simulink model "SC228_TrackedRadarModelUnitTest"  (R2018b)
settings: Solver=VariableStepAuto  StartTime=0.0  StopTime=180  RelTol=1e-3
model workspace (MAT data in the model file):
  E_tracked_bias_stddev_ft = Simulink.Parameter
  E_tracked_bias_stddev_ft.Value = 0
  E_tracked_bias_stddev_ft.DataType = 'auto'
  E_tracked_bias_stddev_ft.Dimensions = [1 1]
  E_tracked_random_stddev_ft = Simulink.Parameter
  E_tracked_random_stddev_ft.Value = 250
  E_tracked_random_stddev_ft.DataType = 'auto'
  E_tracked_random_stddev_ft.Dimensions = [1 1]
  Edot_tracked_bias_stddev_ftps = Simulink.Parameter
  Edot_tracked_bias_stddev_ftps.Value = 0
  Edot_tracked_bias_stddev_ftps.DataType = 'auto'
  Edot_tracked_bias_stddev_ftps.Dimensions = [1 1]
  Edot_tracked_random_stddev_ftps = Simulink.Parameter
  Edot_tracked_random_stddev_ftps.Value = 84.3904928551
  Edot_tracked_random_stddev_ftps.DataType = 'auto'
  Edot_tracked_random_stddev_ftps.Dimensions = [1 1]
  Edot_tracked_tau_s = Simulink.Parameter
  Edot_tracked_tau_s.Value = 0
  Edot_tracked_tau_s.DataType = 'auto'
  Edot_tracked_tau_s.Dimensions = [1 1]
  N_tracked_bias_stddev_ft = Simulink.Parameter
  N_tracked_bias_stddev_ft.Value = 0
  N_tracked_bias_stddev_ft.DataType = 'auto'
  N_tracked_bias_stddev_ft.Dimensions = [1 1]
  N_tracked_random_stddev_ft = 250
  N_tracked_tau_s = Simulink.Parameter
  N_tracked_tau_s.Value = 0
  N_tracked_tau_s.DataType = 'auto'
  N_tracked_tau_s.Dimensions = [1 1]
  Ndot_tracked_bias_stddev_ftps = Simulink.Parameter
  Ndot_tracked_bias_stddev_ftps.Value = 0
  Ndot_tracked_bias_stddev_ftps.DataType = 'auto'
  Ndot_tracked_bias_stddev_ftps.Dimensions = [1 1]
  Ndot_tracked_random_stddev_ftps = Simulink.Parameter
  Ndot_tracked_random_stddev_ftps.Value = 84.3904928551
  Ndot_tracked_random_stddev_ftps.DataType = 'auto'
  Ndot_tracked_random_stddev_ftps.Dimensions = [1 1]
  Ndot_tracked_tau_s = Simulink.Parameter
  Ndot_tracked_tau_s.Value = 0
  Ndot_tracked_tau_s.DataType = 'auto'
  Ndot_tracked_tau_s.Dimensions = [1 1]
  tracked_az_bias_rad = Simulink.Parameter
  tracked_az_bias_rad.Value = 0
  tracked_az_bias_rad.DataType = 'auto'
  tracked_az_bias_rad.Dimensions = [1 1]
  tracked_az_random_stddev_rad = Simulink.Parameter
  tracked_az_random_stddev_rad.Value = 0.0174532925199
  tracked_az_random_stddev_rad.DataType = 'auto'
  tracked_az_random_stddev_rad.Dimensions = [1 1]
  tracked_rng_bias_ft = Simulink.Parameter
  tracked_rng_bias_ft.DataType = 'auto'
  tracked_rng_bias_ft.Dimensions = [0 0]
undefined symbols (not defined in the file or in its folder): ac1dyn_alt0_ft, ac1dyn_con, ac1dyn_lat0_rad, ac1dyn_lon0_rad, ac2dyn_alt0_ft, ac2dyn_con, ac2dyn_lat0_rad, ac2dyn_lon0_rad, ddh_ftps2, dh_ftps, dv_ftps2, e_ft, Edot_ftps, h_ft, hdot_ftps, latLonAltState, n_ft, Ndot_ftps, p_radps, phi_rad, phidot_radps, psi_rad, psidot_radps, q_radps, r_radps, theta_rad, thetadot_radps, uas_rdr_trckd_az_bias_ft, uas_rdr_trckd_az_bias_rad, uas_rdr_trckd_az_random_stddev_rad, uas_rdr_trckd_az_stddev_ft, uas_rdr_trckd_azdot_bias_ftps, uas_rdr_trckd_azdot_stddev_ftps, uas_rdr_trckd_debugMode, uas_rdr_trckd_dt_s, uas_rdr_trckd_el_bias_ft, uas_rdr_trckd_el_bias_rad, uas_rdr_trckd_el_random_stddev_rad, uas_rdr_trckd_el_stddev_ft, uas_rdr_trckd_eldot_bias_ftps, uas_rdr_trckd_eldot_stddev_ftps, uas_rdr_trckd_RCPR_Mode, uas_rdr_trckd_RCPR_Range_ft, uas_rdr_trckd_reported_errorCovRAE, uas_rdr_trckd_rng_bias_ft, uas_rdr_trckd_rng_random_stddev_ft, uas_rdr_trckd_rngdot_bias_ftps, uas_rdr_trckd_rngdot_random_stddev_ftps, uas_rdr_trckd_seed1, uas_rdr_trckd_seed2, uas_rdr_trckd_seed3, uas_rdr_trckd_seed4, uas_rdr_trckd_sns_for_azimuth_deg, uas_rdr_trckd_sns_for_elevation_deg, v_ftps, vdot_fpss
libraries: simulink x17, dspmtrx3 x1
(part 1 of 2)
settings Model: Creator=PE29732  LastModifiedBy=PE29732

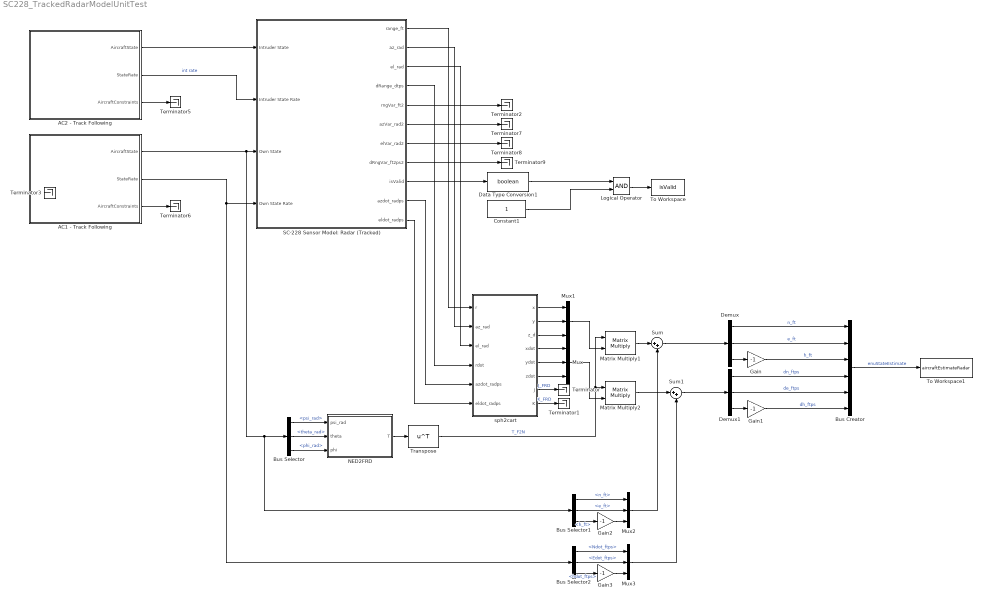
== system SC228_TrackedRadarModelUnitTest ==
  AC1 - Track Following : Subsystem  mask(Basic Aircraft Dynamic Model){ts_dynamics=0.1, lat0_rad=ac1dyn_lat0_rad, lon0_rad=ac1dyn_lon0_rad, alt_ft=ac1dyn_alt0_ft, v_ftps_max=ac1dyn_con.maxAirspeed_ftps, v_ftps_min=ac1dyn_con.minAirspeed_ftps, dv_ftpss_max=ac1dyn_con.maxAcceleration_ftpss, dv_ftpss_min=ac1dyn_con.minAcceleration_ftpss, dh_ftps_max=ac1dyn_con.maxVerticalRate_ftps, dh_ftps_min=ac1dyn_con.minVerticalRate_ftps, q_radps_max=ac1dyn_con.maxPitchRate_radps, phi_rad_max=ac1dyn_con.maxBankAngle_rad, dphi_radps_max=ac1dyn_con.maxRollRate_radps, r_radps_max=ac1dyn_con.maxYawRate_radps, pNUM=ac1dyn_con.dynamicsNumeratorRollRate, pDEN=ac1dyn_con.dynamicsDenominatorRollRate, hNUM=ac1dyn_con.dynamicsNumeratorVerticalRate, hDEN=ac1dyn_con.dynamicsDenominatorVerticalRate, rNUM=ac1dyn_con.dynamicsNumeratorYawRate, rDEN=ac1dyn_con.dynamicsDenominatorYawRate}
      mask prompts: ts_dynamics "Dynamics update parameter"; lat0_rad "Latitude of ENU origin (rad)"; lon0_rad "Longitude of ENU origin (rad)"; alt_ft "Height of ENU origin (ft)"; v_ftps_max "Maximum airspeed (ft/s)"; v_ftps_min "Minimum airspeed (ft/s)"; dv_ftpss_max "Maximum acceleration (ft/s/s)"; dv_ftpss_min "Miniimum acceleration (ft/s/s)"; dh_ftps_max "Maximum vertical rate (ft/s)"; dh_ftps_min "Minimum vertical rate (ft/s)"; q_radps_max "Maximum pitch rate (rad/s)"; phi_rad_max "Maximum bank angle (rad)"; dphi_radps_max "Maximum roll rate (rad/s)"; r_radps_max "Maximum yaw rate (rad/s)"; pNUM "Roll rate discrete dynamics numerator (2x1)"; pDEN "Roll rate discrete dynamics denominator (1x1)"; hNUM "Vertical rate discrete dynamics numerator (2x1)"; hDEN "Vertical rate discrete dynamics denominator (1x1)"; rNUM "Yaw rate discrete dynamics numerator (2x1)"; rDEN "Yaw rate discrete dynamics denominator (1x1)"
      mask help:
      | Propagates the aircraft dynamics using 6DOF equations of motion.
      |
      | The class Simple6DOF can be used to programmatically set the parameters of Basic Aircraft Dynamcis blocks.
      mask Help:
      | Propagates the aircraft dynamics using 6DOF equations of motion.
      | 
      | The class Simple6DOF can be used to programmatically set the parameters of Basic Aircraft Dynamcis blocks.
      mask DialogControl ParameterTabVar0 Prompt: Main
      mask DialogControl ParameterTabVar01 Prompt: Constraints
  AC2 - Track Following : Subsystem  mask(Basic Aircraft Dynamic Model){ts_dynamics=0.1, lat0_rad=ac2dyn_lat0_rad, lon0_rad=ac2dyn_lon0_rad, alt_ft=ac2dyn_alt0_ft, v_ftps_max=ac2dyn_con.maxAirspeed_ftps, v_ftps_min=ac2dyn_con.minAirspeed_ftps, dv_ftpss_max=ac2dyn_con.maxAcceleration_ftpss, dv_ftpss_min=ac2dyn_con.minAcceleration_ftpss, dh_ftps_max=ac2dyn_con.maxVerticalRate_ftps, dh_ftps_min=ac2dyn_con.minVerticalRate_ftps, q_radps_max=ac2dyn_con.maxPitchRate_radps, phi_rad_max=ac2dyn_con.maxBankAngle_rad, dphi_radps_max=ac2dyn_con.maxRollRate_radps, r_radps_max=ac2dyn_con.maxYawRate_radps, pNUM=ac2dyn_con.dynamicsNumeratorRollRate, pDEN=ac2dyn_con.dynamicsDenominatorRollRate, hNUM=ac2dyn_con.dynamicsNumeratorVerticalRate, hDEN=ac2dyn_con.dynamicsDenominatorVerticalRate, rNUM=ac2dyn_con.dynamicsNumeratorYawRate, rDEN=ac2dyn_con.dynamicsDenominatorYawRate}
      mask prompts: ts_dynamics "Dynamics update parameter"; lat0_rad "Latitude of ENU origin (rad)"; lon0_rad "Longitude of ENU origin (rad)"; alt_ft "Height of ENU origin (ft)"; v_ftps_max "Maximum airspeed (ft/s)"; v_ftps_min "Minimum airspeed (ft/s)"; dv_ftpss_max "Maximum acceleration (ft/s/s)"; dv_ftpss_min "Miniimum acceleration (ft/s/s)"; dh_ftps_max "Maximum vertical rate (ft/s)"; dh_ftps_min "Minimum vertical rate (ft/s)"; q_radps_max "Maximum pitch rate (rad/s)"; phi_rad_max "Maximum bank angle (rad)"; dphi_radps_max "Maximum roll rate (rad/s)"; r_radps_max "Maximum yaw rate (rad/s)"; pNUM "Roll rate discrete dynamics numerator (2x1)"; pDEN "Roll rate discrete dynamics denominator (1x1)"; hNUM "Vertical rate discrete dynamics numerator (2x1)"; hDEN "Vertical rate discrete dynamics denominator (1x1)"; rNUM "Yaw rate discrete dynamics numerator (2x1)"; rDEN "Yaw rate discrete dynamics denominator (1x1)"
      mask help:
      | Propagates the aircraft dynamics using 6DOF equations of motion.
      |
      | The class Simple6DOF can be used to programmatically set the parameters of Basic Aircraft Dynamcis blocks.
      mask Help:
      | Propagates the aircraft dynamics using 6DOF equations of motion.
      | 
      | The class Simple6DOF can be used to programmatically set the parameters of Basic Aircraft Dynamcis blocks.
      mask DialogControl ParameterTabVar0 Prompt: Main
      mask DialogControl ParameterTabVar01 Prompt: Constraints
  Bus Creator : BusCreator  Inputs=6  OutDataTypeStr=Bus: StateEstimate
  Bus Selector : BusSelector  OutputSignals=psi_rad,theta_rad,phi_rad
  Bus Selector1 : BusSelector  OutputSignals=n_ft,e_ft,h_ft
  Bus Selector2 : BusSelector  OutputSignals=Ndot_ftps,Edot_ftps,hdot_ftps
  Constant1 : Constant
  Data Type Conversion1 : DataTypeConversion  OutDataTypeStr=boolean
  Demux : Demux  Outputs=3
  Demux1 : Demux  Outputs=3
  Gain{,1..3} (4 alike) : Gain  Gain=-1
  Logical Operator : Logic  AllPortsSameDT=off  OutDataTypeStr=boolean
  Matrix Multiply1 : Product  Multiplication=Matrix(*)
  Matrix Multiply2 : Product  Multiplication=Matrix(*)
  Mux{,1..3} (4 alike) : Mux  Inputs=3
  NED2FRD : MATLAB Function  TreatAsAtomicUnit=on
  SC-228 Sensor Model: Radar (Tracked) : Subsystem  mask(Tracked Surveillance: Radar){dt_s=uas_rdr_trckd_dt_s, lat0_rad=ac1dyn_lat0_rad, lon0_rad=ac1dyn_lon0_rad, alt0_ft=ac1dyn_alt0_ft, sns_for_azimuth_deg=uas_rdr_trckd_sns_for_azimuth_deg, sns_for_elevation_deg=uas_rdr_trckd_sns_for_elevation_deg, debugMode=uas_rdr_trckd_debugMode, rng_random_stddev_ft=uas_rdr_trckd_rng_random_stddev_ft, rng_bias_ft=uas_rdr_trckd_rng_bias_ft, rng_tau_s=0, seed1=uas_rdr_trckd_seed1, RCPR_Mode=uas_rdr_trckd_RCPR_Mode, RCPR_Range_ft=uas_rdr_trckd_RCPR_Range_ft, az_random_stddev_rad=uas_rdr_trckd_az_random_stddev_rad, az_bias_rad=uas_rdr_trckd_az_bias_rad, az_tau_s=0, seed2=uas_rdr_trckd_seed2, el_random_stddev_rad=uas_rdr_trckd_el_random_stddev_rad, el_bias_rad=uas_rdr_trckd_el_bias_rad, el_tau_s=0, seed3=uas_rdr_trckd_seed3, rngdot_random_stddev_ftps=uas_rdr_trckd_rngdot_random_stddev_ftps, rngdot_bias_ftps=uas_rdr_trckd_rngdot_bias_ftps, rngdot_tau_s=0, seed4=uas_rdr_trckd_seed4, covRAE=uas_rdr_trckd_reported_errorCovRAE}
      mask prompts: dt_s "Timestep"; lat0_rad "ENU Origin Latitude"; lon0_rad "ENU Origin Longitude"; alt0_ft "ENU Origin Altitude"; sns_for_azimuth_deg "Field of Regard: Azimuth Limit (deg)"; sns_for_elevation_deg "Field of Regard: Elevation Limit (deg)"; debugMode "Whether to run in debug mode with inifinite detection range"; rng_random_stddev_ft "Range Random Error Standard Deviation"; rng_bias_ft "Range Bias"; rng_tau_s "Correlation Time"; seed1 "Random Seed"; RCPR_Mode "RCPR Mode (1 = minimum range enabled, 0 = not enabled)"; RCPR_Range_ft "RCPR Range (ft)"; az_random_stddev_rad "Azimuth Random Error Standard Deviation"; az_bias_rad "Azimuth Bias"; az_tau_s "Correlation Time"; seed2 "Random Seed"; el_random_stddev_rad "Elevation Random Error Standard Deviation"; el_bias_rad "Elevation Bias"; el_tau_s "Correlation Time"; seed3 "Random Seed"; rngdot_random_stddev_ftps "Range Rate Random Error Standard Deviation"; rngdot_bias_ftps "Range Rate Bias"; rngdot_tau_s "Correlation Time"; seed4 "Random Seed"; covRAE "Error Covariance"
      mask help: Additive noise model of an on-board radar
      mask Help:
      | Additive noise model of an on-board radar.  Independent noise is added to
      | each of range, azimuth, elevation and their rates.  Noise is colored using
      | weights determined by time constant parameters.
      | 
      | Output takes the form of a AircraftEstimate data bus and a 6x6 error covariance
      | matrix in North-East-Down.  State order in error covariance output is
      | [ posN posE posD velN velE velD ].
      | 
      | Model originally developed for USAF Common ABSAA Program Nov 2013
      mask DialogControl ParameterTabVar0 Prompt: Tab
      mask DialogControl ParameterTabVar01 Prompt: Range
      mask DialogControl ParameterTabVar012 Prompt: Azimuth
      mask DialogControl ParameterTabVar0123 Prompt: Elevation
      mask DialogControl ParameterTabVar01234 Prompt: Range rate
      mask DialogControl ParameterTabVar01234567 Prompt: Covariance
  Sum : Sum  Inputs=|++
  Sum1 : Sum  Inputs=|++
  Terminator{,1..3,5..9} (9 alike) : Terminator
  To Workspace : ToWorkspace  VariableName=isValid  SaveFormat=Timeseries  SampleTime=-1
  To Workspace1 : ToWorkspace  VariableName=aircraftEstimateRadar  SaveFormat=Timeseries  SampleTime=-1
  Transpose : Math  Operator=transpose  SaturateOnIntegerOverflow=on
  sph2cart : MATLAB Function  TreatAsAtomicUnit=on
  wires:
  AC1 - Track Following/2(StateRate) -> Bus Selector2/1, SC-228 Sensor Model: Radar (Tracked)/4(Own State Rate)
  Bus Selector2/1 -> Mux3/1  "<Ndot_ftps>"
  Data Type Conversion1/1 -> Logical Operator/1
  SC-228 Sensor Model: Radar (Tracked)/10(azdot_radps) -> sph2cart/5(azdot_radps)
  sph2cart/1(x) -> Mux1/1
  Bus Creator/1 -> To Workspace1/1  "enuStateEstimate"
  AC2 - Track Following/1(AircraftState) -> SC-228 Sensor Model: Radar (Tracked)/1(Intruder State)
  Gain1/1 -> Bus Creator/6  "dh_ftps"
  SC-228 Sensor Model: Radar (Tracked)/2(az_rad) -> sph2cart/2(az_rad)
  Gain/1 -> Bus Creator/3  "h_ft"
  Bus Selector1/3 -> Gain2/1  "<h_ft>"
  Bus Selector1/1 -> Mux2/1  "<n_ft>"
  Mux/1 -> Matrix Multiply2/2
  sph2cart/6(zdot) -> Mux/3
  Demux1/1 -> Bus Creator/4  "dn_ftps"
  SC-228 Sensor Model: Radar (Tracked)/7(elVar_rad2) -> Terminator8/1
  SC-228 Sensor Model: Radar (Tracked)/3(el_rad) -> sph2cart/3(el_rad)
  Demux/2 -> Bus Creator/2  "e_ft"
  sph2cart/3(z_d) -> Mux1/3
  sph2cart/5(ydot) -> Mux/2
  Sum1/1 -> Demux1/1
  SC-228 Sensor Model: Radar (Tracked)/9(isValid) -> Data Type Conversion1/1
  Sum/1 -> Demux/1
  Demux1/2 -> Bus Creator/5  "de_ftps"
  sph2cart/2(y) -> Mux1/2
  Bus Selector2/2 -> Mux3/2  "<Edot_ftps>"
  Demux/1 -> Bus Creator/1  "n_ft"
  Bus Selector/1 -> NED2FRD/1(psi_rad)  "<psi_rad>"
  Demux/3 -> Gain/1
  Bus Selector1/2 -> Mux2/2  "<e_ft>"
  SC-228 Sensor Model: Radar (Tracked)/1(range_ft) -> sph2cart/1(r)
  SC-228 Sensor Model: Radar (Tracked)/11(eldot_radps) -> sph2cart/6(eldot_radps)
  SC-228 Sensor Model: Radar (Tracked)/4(dRange_dtps) -> sph2cart/4(rdot)
  NED2FRD/1(T) -> Transpose/1
  sph2cart/8(K) -> Terminator1/1  "K_FRD"
  Bus Selector/2 -> NED2FRD/2(theta)  "<theta_rad>"
  Matrix Multiply1/1 -> Sum/1
  AC1 - Track Following/1(AircraftState) -> Bus Selector1/1, Bus Selector/1, SC-228 Sensor Model: Radar (Tracked)/3(Own State)
  Gain2/1 -> Mux2/3
  sph2cart/4(xdot) -> Mux/1
  Mux1/1 -> Matrix Multiply1/2
  sph2cart/7(J) -> Terminator/1  "J_FRD"
  Matrix Multiply2/1 -> Sum1/1
  Mux2/1 -> Sum/2
  Bus Selector/3 -> NED2FRD/3(phi)  "<phi_rad>"
  Transpose/1 -> Matrix Multiply1/1, Matrix Multiply2/1  "T_F2N"
  Demux1/3 -> Gain1/1
  Constant1/1 -> Logical Operator/2
  Mux3/1 -> Sum1/2
  Logical Operator/1 -> To Workspace/1
  AC2 - Track Following/3(AircraftConstraints) -> Terminator5/1
  AC2 - Track Following/2(StateRate) -> SC-228 Sensor Model: Radar (Tracked)/2(Intruder State Rate)  "int rate"
  AC1 - Track Following/3(AircraftConstraints) -> Terminator6/1
  SC-228 Sensor Model: Radar (Tracked)/6(azVar_rad2) -> Terminator7/1
  SC-228 Sensor Model: Radar (Tracked)/8(dRngVar_ft2ps2) -> Terminator9/1
  SC-228 Sensor Model: Radar (Tracked)/5(rngVar_ft2) -> Terminator2/1
  Bus Selector2/3 -> Gain3/1  "<hdot_ftps>"
  Gain3/1 -> Mux3/3

== system SC228_TrackedRadarModelUnitTest/AC1 - Track Following ==
  Follow Trajectory : Subsystem  mask(Follow Trajectory){trajfile=traj1.mat}
      mask prompts: trajfile "Trajectory File Name:"
      mask help: Reads trajectory data (North-East-Altitude position and velocity) from specified file. Computes other state variables to follow that trajectory. Ouptuts AircraftState and AircraftStateRate buses.
      mask init:
      | set_param( [ gcb '/Get Trajectory Data/From File' ], 'Filename', trajfile )
  Performance_constraints : Subsystem
  Rate Transition : RateTransition  OutPortSampleTime=0.1
  AircraftState : Outport  OutDataTypeStr=Bus: AircraftState
  StateRate : Outport  Port=2  OutDataTypeStr=Bus: AircraftStateRate
  AircraftConstraints : Outport  Port=3  OutDataTypeStr=Bus: AircraftConstraints
  wires:
  Follow Trajectory/2(State Rate) -> Rate Transition/1
  Follow Trajectory/1(State) -> AircraftState/1
  Performance_constraints/1(AircraftConstraints) -> Follow Trajectory/1(Constraints), AircraftConstraints/1
  Rate Transition/1 -> StateRate/1

== system SC228_TrackedRadarModelUnitTest/AC2 - Track Following ==
  Follow Trajectory : Subsystem  mask(Follow Trajectory){trajfile=traj2.mat}
      mask prompts: trajfile "Trajectory File Name:"
      mask help: Reads trajectory data (North-East-Altitude position and velocity) from specified file. Computes other state variables to follow that trajectory. Ouptuts AircraftState and AircraftStateRate buses.
      mask init:
      | set_param( [ gcb '/Get Trajectory Data/From File' ], 'Filename', trajfile )
  Performance_constraints : Subsystem
  Rate Transition : RateTransition  OutPortSampleTime=0.1
  AircraftState : Outport  OutDataTypeStr=Bus: AircraftState
  StateRate : Outport  Port=2  OutDataTypeStr=Bus: AircraftStateRate
  AircraftConstraints : Outport  Port=3  OutDataTypeStr=Bus: AircraftConstraints
  wires:
  Follow Trajectory/2(State Rate) -> Rate Transition/1
  Follow Trajectory/1(State) -> AircraftState/1
  Performance_constraints/1(AircraftConstraints) -> Follow Trajectory/1(Constraints), AircraftConstraints/1
  Rate Transition/1 -> StateRate/1

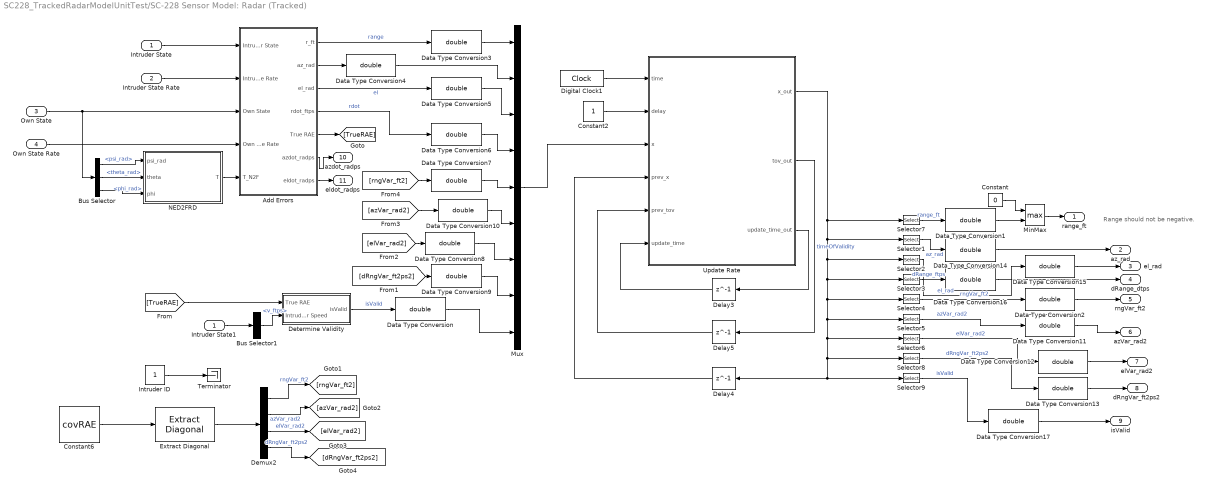
== system SC228_TrackedRadarModelUnitTest/SC-228 Sensor Model: Radar (Tracked) ==
  note: Range should not be negative.
  Intruder State : Inport  OutDataTypeStr=Bus: AircraftState
  Intruder State Rate : Inport  Port=2  OutDataTypeStr=Bus: AircraftStateRate
  Own State : Inport  Port=3  OutDataTypeStr=Bus: AircraftState
  Own State Rate : Inport  Port=4  OutDataTypeStr=Bus: AircraftStateRate
  Add Errors : Subsystem
  Bus Selector : BusSelector  OutputSignals=psi_rad,theta_rad,phi_rad
  Bus Selector1 : BusSelector  OutputSignals=v_ftps
  Constant : Constant  Value=0
  Constant2 : Constant
  Constant6 : Constant  Value=covRAE
  Data Type Conversion{,1..17} (18 alike) : DataTypeConversion  OutDataTypeStr=double
  Delay3 : Delay  DelayLength=1  InitialCondition=1
  Delay4 : Delay  DelayLength=1  InitialCondition=0
  Delay5 : Delay  DelayLength=1  InitialCondition=0
  Demux2 : Demux
  Determine Validity : Subsystem
  Digital Clock1 : DigitalClock  SampleTime=0.1
  Extract Diagonal : dspmtrx3/Extract Diagonal
      settings: SourceProductName=DSP System Toolbox  SourceProductBaseCode=DS
  Intruder ID : Constant
  Intruder State1 : InportShadow  OutDataTypeStr=Bus: AircraftState
  MinMax : MinMax  Function=max  Inputs=2
  Mux : Mux  Inputs=9
  NED2FRD : MATLAB Function  TreatAsAtomicUnit=on
  Selector1 : Selector  InputPortWidth=9  IndexOptions=Index vector (dialog)  Indices=[2]  OutputSizes=1
  Selector2 : Selector  InputPortWidth=9  IndexOptions=Index vector (dialog)  Indices=[3]  OutputSizes=1
  Selector3 : Selector  InputPortWidth=9  IndexOptions=Index vector (dialog)  Indices=[4]  OutputSizes=1
  Selector4 : Selector  InputPortWidth=9  IndexOptions=Index vector (dialog)  Indices=[5]  OutputSizes=1
  Selector5 : Selector  InputPortWidth=9  IndexOptions=Index vector (dialog)  Indices=[6]  OutputSizes=1
  Selector6 : Selector  InputPortWidth=9  IndexOptions=Index vector (dialog)  Indices=[7]  OutputSizes=1
  Selector7 : Selector  InputPortWidth=9  IndexOptions=Index vector (dialog)  Indices=[1]  OutputSizes=1
  Selector8 : Selector  InputPortWidth=9  IndexOptions=Index vector (dialog)  Indices=[8]  OutputSizes=1
  Selector9 : Selector  InputPortWidth=9  IndexOptions=Index vector (dialog)  Indices=[9]  OutputSizes=1
  Terminator : Terminator
  Update Rate : MATLAB Function  TreatAsAtomicUnit=on
  range_ft : Outport
  az_rad : Outport  Port=2
  el_rad : Outport  Port=3
  dRange_dtps : Outport  Port=4
  rngVar_ft2 : Outport  Port=5
  azVar_rad2 : Outport  Port=6
  elVar_rad2 : Outport  Port=7
  dRngVar_ft2ps2 : Outport  Port=8
  isValid : Outport  Port=9
  azdot_radps : Outport  Port=10
  eldot_radps : Outport  Port=11
  wires:
  Data Type Conversion13/1 -> dRngVar_ft2ps2/1
  Data Type Conversion12/1 -> elVar_rad2/1
  Data Type Conversion11/1 -> azVar_rad2/1
  Data Type Conversion7/1 -> Mux/5
  Data Type Conversion10/1 -> Mux/6
  Data Type Conversion9/1 -> Mux/8
  [dRngVar_ft2ps2] -> Data Type Conversion9/1
  Data Type Conversion8/1 -> Mux/7
  [rngVar_ft2] -> Data Type Conversion7/1
  Data Type Conversion6/1 -> Mux/4
  Data Type Conversion5/1 -> Mux/3
  Data Type Conversion4/1 -> Mux/2
  Data Type Conversion3/1 -> Mux/1
  Data Type Conversion2/1 -> rngVar_ft2/1
  Data Type Conversion1/1 -> MinMax/2
  Add Errors/4(rdot_ftps) -> Data Type Conversion6/1  "rdot"
  Add Errors/3(el_rad) -> Data Type Conversion5/1  "el"
  Bus Selector/3 -> NED2FRD/3(phi)  "<phi_rad>"
  Own State/1 -> Bus Selector/1, Add Errors/3(Own State)
  Bus Selector/1 -> NED2FRD/1(psi_rad)  "<psi_rad>"
  Bus Selector/2 -> NED2FRD/2(theta)  "<theta_rad>"
  Add Errors/1(r_ft) -> Data Type Conversion3/1  "range"
  NED2FRD/1(T) -> Add Errors/5(T_N2F)
  Own State Rate/1 -> Add Errors/4(Own State Rate)
  Add Errors/5(True RAE) -> [TrueRAE]
  [TrueRAE] -> Determine Validity/1(True RAE)
  Intruder ID/1 -> Terminator/1
  Determine Validity/1(isValid) -> Data Type Conversion/1  "isValid"
  Digital Clock1/1 -> Update Rate/1(time)
  Constant2/1 -> Update Rate/2(delay)
  [azVar_rad2] -> Data Type Conversion10/1
  [elVar_rad2] -> Data Type Conversion8/1
  Mux/1 -> Update Rate/3(x)
  Delay5/1 -> Update Rate/5(prev_tov)
  Update Rate/2(tov_out) -> Delay5/1  "timeOfValidity"
  Delay3/1 -> Update Rate/6(update_time)
  Delay4/1 -> Update Rate/4(prev_x)
  Update Rate/3(update_time_out) -> Delay3/1
  Update Rate/1(x_out) -> Selector2/1, Selector3/1, Selector4/1, Selector5/1, Selector6/1, Selector8/1, Selector9/1, Delay4/1, Selector1/1, Selector7/1
  Selector7/1 -> Data Type Conversion1/1  "range_ft"
  Selector1/1 -> Data Type Conversion14/1  "az_rad"
  Selector2/1 -> Data Type Conversion15/1  "el_rad"
  Selector3/1 -> Data Type Conversion16/1  "dRange_ftps"
  Selector4/1 -> Data Type Conversion2/1  "rngVar_ft2"
  Selector5/1 -> Data Type Conversion11/1  "azVar_rad2"
  Selector6/1 -> Data Type Conversion12/1  "elVar_rad2"
  Selector8/1 -> Data Type Conversion13/1  "dRngVar_ft2ps2"
  Selector9/1 -> Data Type Conversion17/1  "isValid"
  Intruder State1/1 -> Bus Selector1/1
  Bus Selector1/1 -> Determine Validity/2(Intruder Speed)  "<v_ftps>"
  Constant6/1 -> Extract Diagonal/1
  Extract Diagonal/1 -> Demux2/1
  Demux2/1 -> [rngVar_ft2]  "rngVar_ft2"
  Demux2/2 -> [azVar_rad2]  "azVar_rad2"
  Demux2/3 -> [elVar_rad2]  "elVar_rad2"
  Demux2/4 -> [dRngVar_ft2ps2]  "dRngVar_ft2ps2"
  Data Type Conversion/1 -> Mux/9
  MinMax/1 -> range_ft/1
  Constant/1 -> MinMax/1
  Data Type Conversion14/1 -> az_rad/1
  Data Type Conversion15/1 -> el_rad/1
  Data Type Conversion16/1 -> dRange_dtps/1
  Data Type Conversion17/1 -> isValid/1
  Add Errors/6(azdot_radps) -> azdot_radps/1
  Add Errors/7(eldot_radps) -> eldot_radps/1
  Intruder State Rate/1 -> Add Errors/2(Intruder State Rate)
  Intruder State/1 -> Add Errors/1(Intruder State)
  Add Errors/2(az_rad) -> Data Type Conversion4/1

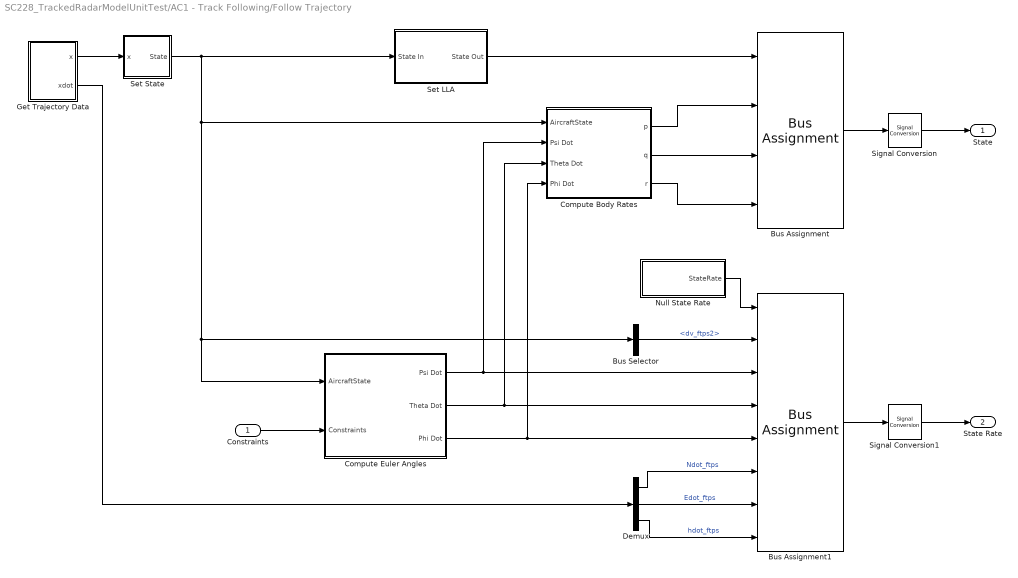
== system SC228_TrackedRadarModelUnitTest/AC1 - Track Following/Follow Trajectory ==
  Constraints : Inport
  Bus Assignment : BusAssignment  AssignedSignals=p_radps,q_radps,r_radps
  Bus Assignment1 : BusAssignment  AssignedSignals=vdot_fpss,psidot_radps,thetadot_radps,phidot_radps,Ndot_ftps,Edot_ftps,hdot_ftps
  Bus Selector : BusSelector  OutputSignals=dv_ftps2
  Compute Body Rates : Subsystem
  Compute Euler Angles : Subsystem
  Demux : Demux  Outputs=3
  Get Trajectory Data : Subsystem
  Null State Rate : Subsystem
  "Set LLA " : Subsystem  mask{lat0=lat0_rad, lon0=lon0_rad, h0=alt_ft}
      mask prompts: lat0 "ENU latitude origin (rad)"; lon0 "ENU longitude origin (rad)"; h0 "ENU altitude origin (ft)"
  Set State : Subsystem
  Signal Conversion : SignalConversion  OverrideOpt=off
  Signal Conversion1 : SignalConversion  OverrideOpt=off
  State : Outport
  State Rate : Outport  Port=2
  wires:
  Signal Conversion1/1 -> State Rate/1
  Bus Selector/1 -> Bus Assignment1/2  "<dv_ftps2>"
  Compute Euler Angles/3("Phi Dot ") -> Bus Assignment1/5, Compute Body Rates/4(Phi Dot)
  Compute Euler Angles/1(Psi Dot) -> Bus Assignment1/3, Compute Body Rates/2(Psi Dot)
  Demux/3 -> Bus Assignment1/8  "hdot_ftps"
  Null State Rate/1(StateRate) -> Bus Assignment1/1
  Get Trajectory Data/2(xdot) -> Demux/1
  Compute Body Rates/3(r) -> Bus Assignment/4
  Compute Body Rates/2(q) -> Bus Assignment/3
  Compute Body Rates/1(p) -> Bus Assignment/2
  Demux/1 -> Bus Assignment1/6  "Ndot_ftps"
  Demux/2 -> Bus Assignment1/7  "Edot_ftps"
  Compute Euler Angles/2(Theta Dot) -> Bus Assignment1/4, Compute Body Rates/3(Theta Dot)
  Signal Conversion/1 -> State/1
  "Set LLA "/1(State Out) -> Bus Assignment/1
  Bus Assignment/1 -> Signal Conversion/1
  Bus Assignment1/1 -> Signal Conversion1/1
  Set State/1(State) -> Compute Body Rates/1(AircraftState), Compute Euler Angles/1(AircraftState), Bus Selector/1, "Set LLA "/1(State In)
  Constraints/1 -> Compute Euler Angles/2(Constraints)
  Get Trajectory Data/1(x) -> Set State/1(x)

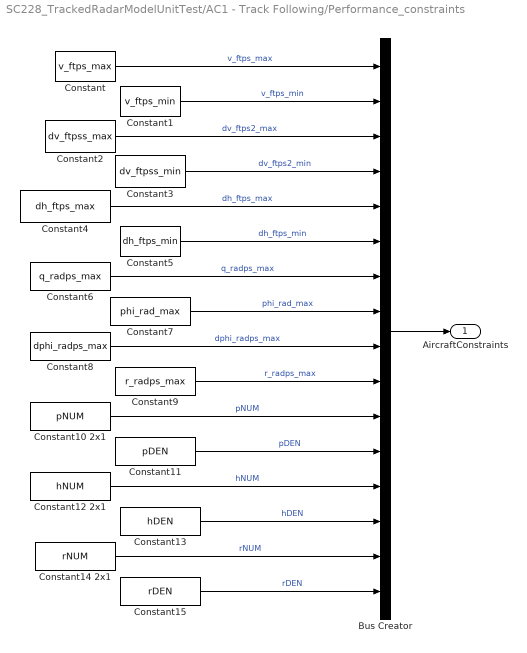
== system SC228_TrackedRadarModelUnitTest/AC1 - Track Following/Performance_constraints ==
  Bus Creator : BusCreator  Inputs=16
  Constant : Constant  Value=v_ftps_max
  Constant1 : Constant  Value=v_ftps_min
  Constant10 2x1 : Constant  Value=pNUM
  Constant11 : Constant  Value=pDEN
  Constant12 2x1 : Constant  Value=hNUM
  Constant13 : Constant  Value=hDEN
  Constant14 2x1 : Constant  Value=rNUM
  Constant15 : Constant  Value=rDEN
  Constant2 : Constant  Value=dv_ftpss_max
  Constant3 : Constant  Value=dv_ftpss_min
  Constant4 : Constant  Value=dh_ftps_max
  Constant5 : Constant  Value=dh_ftps_min
  Constant6 : Constant  Value=q_radps_max
  Constant7 : Constant  Value=phi_rad_max
  Constant8 : Constant  Value=dphi_radps_max
  Constant9 : Constant  Value=r_radps_max
  AircraftConstraints : Outport  OutDataTypeStr=Bus: AircraftConstraints
  wires:
  Constant10 2x1/1 -> Bus Creator/11  "pNUM"
  Constant12 2x1/1 -> Bus Creator/13  "hNUM"
  Constant14 2x1/1 -> Bus Creator/15  "rNUM"
  Constant8/1 -> Bus Creator/9  "dphi_radps_max"
  Constant7/1 -> Bus Creator/8  "phi_rad_max"
  Constant6/1 -> Bus Creator/7  "q_radps_max"
  Constant5/1 -> Bus Creator/6  "dh_ftps_min"
  Constant4/1 -> Bus Creator/5  "dh_ftps_max"
  Constant3/1 -> Bus Creator/4  "dv_ftps2_min"
  Constant2/1 -> Bus Creator/3  "dv_ftps2_max"
  Constant1/1 -> Bus Creator/2  "v_ftps_min"
  Constant/1 -> Bus Creator/1  "v_ftps_max"
  Bus Creator/1 -> AircraftConstraints/1
  Constant15/1 -> Bus Creator/16  "rDEN"
  Constant13/1 -> Bus Creator/14  "hDEN"
  Constant11/1 -> Bus Creator/12  "pDEN"
  Constant9/1 -> Bus Creator/10  "r_radps_max"

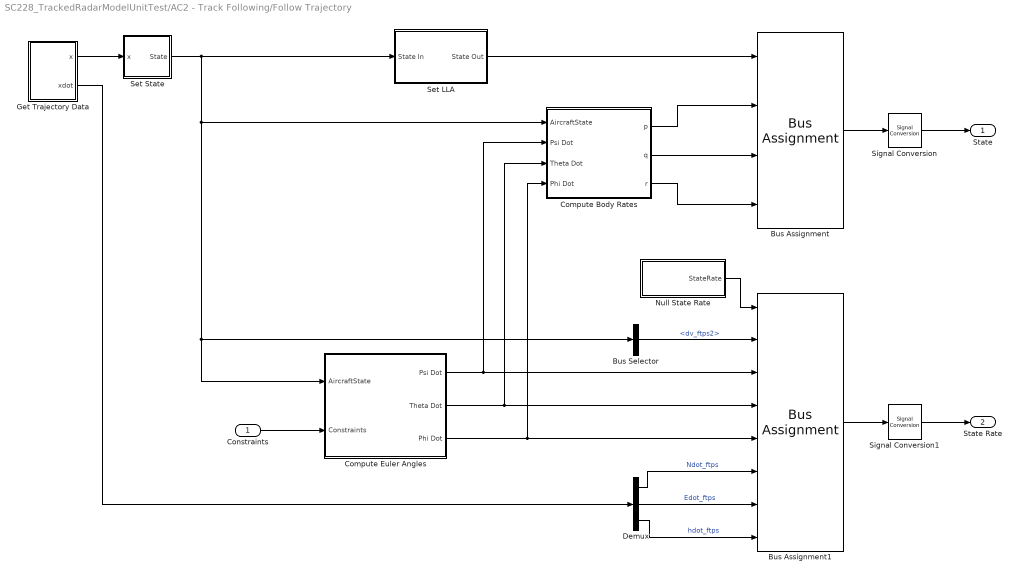
== system SC228_TrackedRadarModelUnitTest/AC2 - Track Following/Follow Trajectory ==
  Constraints : Inport
  Bus Assignment : BusAssignment  AssignedSignals=p_radps,q_radps,r_radps
  Bus Assignment1 : BusAssignment  AssignedSignals=vdot_fpss,psidot_radps,thetadot_radps,phidot_radps,Ndot_ftps,Edot_ftps,hdot_ftps
  Bus Selector : BusSelector  OutputSignals=dv_ftps2
  Compute Body Rates : Subsystem
  Compute Euler Angles : Subsystem
  Demux : Demux  Outputs=3
  Get Trajectory Data : Subsystem
  Null State Rate : Subsystem
  "Set LLA " : Subsystem  mask{lat0=lat0_rad, lon0=lon0_rad, h0=alt_ft}
      mask prompts: lat0 "ENU latitude origin (rad)"; lon0 "ENU longitude origin (rad)"; h0 "ENU altitude origin (ft)"
  Set State : Subsystem
  Signal Conversion : SignalConversion  OverrideOpt=off
  Signal Conversion1 : SignalConversion  OverrideOpt=off
  State : Outport
  State Rate : Outport  Port=2
  wires:
  Signal Conversion1/1 -> State Rate/1
  Bus Selector/1 -> Bus Assignment1/2  "<dv_ftps2>"
  Compute Euler Angles/3("Phi Dot ") -> Bus Assignment1/5, Compute Body Rates/4(Phi Dot)
  Compute Euler Angles/1(Psi Dot) -> Bus Assignment1/3, Compute Body Rates/2(Psi Dot)
  Demux/3 -> Bus Assignment1/8  "hdot_ftps"
  Null State Rate/1(StateRate) -> Bus Assignment1/1
  Get Trajectory Data/2(xdot) -> Demux/1
  Compute Body Rates/3(r) -> Bus Assignment/4
  Compute Body Rates/2(q) -> Bus Assignment/3
  Compute Body Rates/1(p) -> Bus Assignment/2
  Demux/1 -> Bus Assignment1/6  "Ndot_ftps"
  Demux/2 -> Bus Assignment1/7  "Edot_ftps"
  Compute Euler Angles/2(Theta Dot) -> Bus Assignment1/4, Compute Body Rates/3(Theta Dot)
  Signal Conversion/1 -> State/1
  "Set LLA "/1(State Out) -> Bus Assignment/1
  Bus Assignment/1 -> Signal Conversion/1
  Bus Assignment1/1 -> Signal Conversion1/1
  Set State/1(State) -> Compute Body Rates/1(AircraftState), Compute Euler Angles/1(AircraftState), Bus Selector/1, "Set LLA "/1(State In)
  Constraints/1 -> Compute Euler Angles/2(Constraints)
  Get Trajectory Data/1(x) -> Set State/1(x)

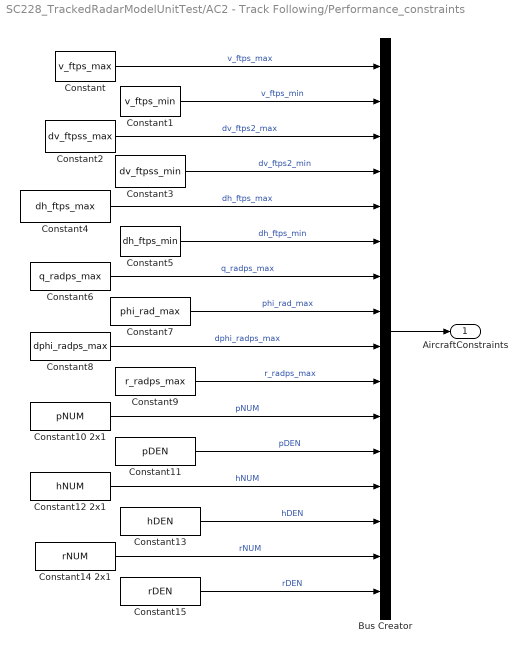
== system SC228_TrackedRadarModelUnitTest/AC2 - Track Following/Performance_constraints ==
  Bus Creator : BusCreator  Inputs=16
  Constant : Constant  Value=v_ftps_max
  Constant1 : Constant  Value=v_ftps_min
  Constant10 2x1 : Constant  Value=pNUM
  Constant11 : Constant  Value=pDEN
  Constant12 2x1 : Constant  Value=hNUM
  Constant13 : Constant  Value=hDEN
  Constant14 2x1 : Constant  Value=rNUM
  Constant15 : Constant  Value=rDEN
  Constant2 : Constant  Value=dv_ftpss_max
  Constant3 : Constant  Value=dv_ftpss_min
  Constant4 : Constant  Value=dh_ftps_max
  Constant5 : Constant  Value=dh_ftps_min
  Constant6 : Constant  Value=q_radps_max
  Constant7 : Constant  Value=phi_rad_max
  Constant8 : Constant  Value=dphi_radps_max
  Constant9 : Constant  Value=r_radps_max
  AircraftConstraints : Outport  OutDataTypeStr=Bus: AircraftConstraints
  wires:
  Constant10 2x1/1 -> Bus Creator/11  "pNUM"
  Constant12 2x1/1 -> Bus Creator/13  "hNUM"
  Constant14 2x1/1 -> Bus Creator/15  "rNUM"
  Constant8/1 -> Bus Creator/9  "dphi_radps_max"
  Constant7/1 -> Bus Creator/8  "phi_rad_max"
  Constant6/1 -> Bus Creator/7  "q_radps_max"
  Constant5/1 -> Bus Creator/6  "dh_ftps_min"
  Constant4/1 -> Bus Creator/5  "dh_ftps_max"
  Constant3/1 -> Bus Creator/4  "dv_ftps2_min"
  Constant2/1 -> Bus Creator/3  "dv_ftps2_max"
  Constant1/1 -> Bus Creator/2  "v_ftps_min"
  Constant/1 -> Bus Creator/1  "v_ftps_max"
  Bus Creator/1 -> AircraftConstraints/1
  Constant15/1 -> Bus Creator/16  "rDEN"
  Constant13/1 -> Bus Creator/14  "hDEN"
  Constant11/1 -> Bus Creator/12  "pDEN"
  Constant9/1 -> Bus Creator/10  "r_radps_max"

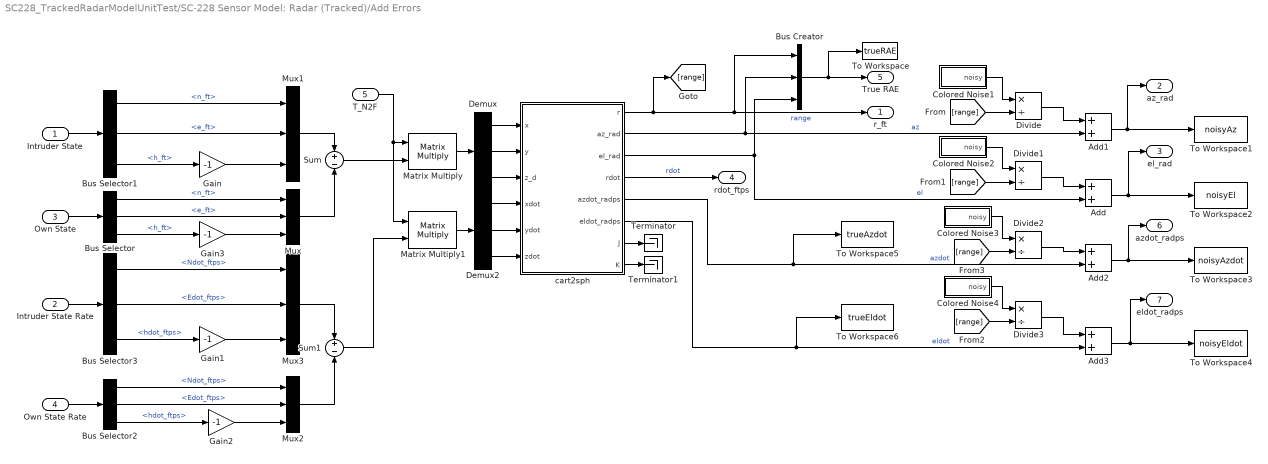
== system SC228_TrackedRadarModelUnitTest/SC-228 Sensor Model: Radar (Tracked)/Add Errors ==
  Intruder State : Inport  OutDataTypeStr=Bus: AircraftState
  Intruder State Rate : Inport  Port=2  OutDataTypeStr=Bus: AircraftStateRate
  Own State : Inport  Port=3  OutDataTypeStr=Bus: AircraftState
  Own State Rate : Inport  Port=4  OutDataTypeStr=Bus: AircraftStateRate
  T_N2F : Inport  Port=5
  Add{,1..3} (4 alike) : Sum
  Bus Creator : BusCreator  Inputs=3
  Bus Selector : BusSelector  OutputSignals=n_ft,e_ft,h_ft
  Bus Selector1 : BusSelector  OutputSignals=n_ft,e_ft,h_ft
  Bus Selector2 : BusSelector  OutputSignals=Ndot_ftps,Edot_ftps,hdot_ftps
  Bus Selector3 : BusSelector  OutputSignals=Ndot_ftps,Edot_ftps,hdot_ftps
  Colored Noise1 : Subsystem  AncestorBlock=Radar_Block/SC-228 Sensor Model: Radar/Add Errors/Colored Noise2  mask(Colored Noise){sig=uas_rdr_trckd_az_stddev_ft, bias=uas_rdr_trckd_az_bias_ft, tau=0, dt=dt_s, seed=seed1}
      mask prompts: sig "Random error standard deviation"; bias "Bias error"; tau "Correlation time"; dt "Track update time"; seed "Random Seed"
      mask help: Generates a noisy state variable estimate using the ABSAA colored noise model. Set correlation time to zero for white noise.
      mask Help:
      | Generates a noisy state variable estimate using the AF Common ABSAA error
      | model.  Time correlation of the error is defined by an exponential decay
      | of K = exp(-tau/dt), where tau is the correlation time and dt is the time
      | between track updates.  The track error at time t is then:
      | 
      |     err(t) = K*err(t-1) + N(0,(1-K^2)*sig^2) + bias
      | 
      | where N(x,y) is a Gaussian noise process with mean x and variance y and
      | with random number generator seeded with the integer 'seed'.
      | 
      | The random noise process must be initialized with an error drawn from
      | N(0,sig^2).
      | 
      | The noise model can be used to produce white noise by setting tau to zero.
  Colored Noise2 : Subsystem  AncestorBlock=Radar_Block/SC-228 Sensor Model: Radar/Add Errors/Colored Noise3  mask(Colored Noise){sig=uas_rdr_trckd_el_stddev_ft, bias=uas_rdr_trckd_el_bias_ft, tau=0, dt=dt_s, seed=seed2}
      mask prompts: sig "Random error standard deviation"; bias "Bias error"; tau "Correlation time"; dt "Track update time"; seed "Random Seed"
      mask help: Generates a noisy state variable estimate using the ABSAA colored noise model. Set correlation time to zero for white noise.
      mask Help:
      | Generates a noisy state variable estimate using the AF Common ABSAA error
      | model.  Time correlation of the error is defined by an exponential decay
      | of K = exp(-tau/dt), where tau is the correlation time and dt is the time
      | between track updates.  The track error at time t is then:
      | 
      |     err(t) = K*err(t-1) + N(0,(1-K^2)*sig^2) + bias
      | 
      | where N(x,y) is a Gaussian noise process with mean x and variance y and
      | with random number generator seeded with the integer 'seed'.
      | 
      | The random noise process must be initialized with an error drawn from
      | N(0,sig^2).
      | 
      | The noise model can be used to produce white noise by setting tau to zero.
  Colored Noise3 : Subsystem  AncestorBlock=Radar_Block/SC-228 Sensor Model: Radar/Add Errors/Colored Noise3  mask(Colored Noise){sig=uas_rdr_trckd_azdot_stddev_ftps, bias=uas_rdr_trckd_azdot_bias_ftps, tau=0, dt=dt_s, seed=seed3}
      mask prompts: sig "Random error standard deviation"; bias "Bias error"; tau "Correlation time"; dt "Track update time"; seed "Random Seed"
      mask help: Generates a noisy state variable estimate using the ABSAA colored noise model. Set correlation time to zero for white noise.
      mask Help:
      | Generates a noisy state variable estimate using the AF Common ABSAA error
      | model.  Time correlation of the error is defined by an exponential decay
      | of K = exp(-tau/dt), where tau is the correlation time and dt is the time
      | between track updates.  The track error at time t is then:
      | 
      |     err(t) = K*err(t-1) + N(0,(1-K^2)*sig^2) + bias
      | 
      | where N(x,y) is a Gaussian noise process with mean x and variance y and
      | with random number generator seeded with the integer 'seed'.
      | 
      | The random noise process must be initialized with an error drawn from
      | N(0,sig^2).
      | 
      | The noise model can be used to produce white noise by setting tau to zero.
  Colored Noise4 : Subsystem  AncestorBlock=Radar_Block/SC-228 Sensor Model: Radar/Add Errors/Colored Noise3  mask(Colored Noise){sig=uas_rdr_trckd_eldot_stddev_ftps, bias=uas_rdr_trckd_eldot_bias_ftps, tau=0, dt=dt_s, seed=seed4}
      mask prompts: sig "Random error standard deviation"; bias "Bias error"; tau "Correlation time"; dt "Track update time"; seed "Random Seed"
      mask help: Generates a noisy state variable estimate using the ABSAA colored noise model. Set correlation time to zero for white noise.
      mask Help:
      | Generates a noisy state variable estimate using the AF Common ABSAA error
      | model.  Time correlation of the error is defined by an exponential decay
      | of K = exp(-tau/dt), where tau is the correlation time and dt is the time
      | between track updates.  The track error at time t is then:
      | 
      |     err(t) = K*err(t-1) + N(0,(1-K^2)*sig^2) + bias
      | 
      | where N(x,y) is a Gaussian noise process with mean x and variance y and
      | with random number generator seeded with the integer 'seed'.
      | 
      | The random noise process must be initialized with an error drawn from
      | N(0,sig^2).
      | 
      | The noise model can be used to produce white noise by setting tau to zero.
  Demux : Demux  Outputs=3
  Demux2 : Demux  Outputs=3
  Divide{,1..3} (4 alike) : Product  Inputs=*/
  Gain{,1..3} (4 alike) : Gain  Gain=-1
  Matrix Multiply : Product  Multiplication=Matrix(*)
  Matrix Multiply1 : Product  Multiplication=Matrix(*)
  Mux{,1..3} (4 alike) : Mux  Inputs=3
  Sum : Sum  Inputs=+-
  Sum1 : Sum  Inputs=+-
  Terminator : Terminator
  Terminator1 : Terminator
  To Workspace : ToWorkspace  VariableName=trueRAE  SaveFormat=Timeseries  SampleTime=-1
  To Workspace1 : ToWorkspace  VariableName=noisyAz  SaveFormat=Timeseries  SampleTime=-1
  To Workspace2 : ToWorkspace  VariableName=noisyEl  SaveFormat=Timeseries  SampleTime=-1
  To Workspace3 : ToWorkspace  VariableName=noisyAzdot  SaveFormat=Timeseries  SampleTime=-1
  To Workspace4 : ToWorkspace  VariableName=noisyEldot  SaveFormat=Timeseries  SampleTime=-1
  To Workspace5 : ToWorkspace  VariableName=trueAzdot  SaveFormat=Timeseries  SampleTime=-1
  To Workspace6 : ToWorkspace  VariableName=trueEldot  SaveFormat=Timeseries  SampleTime=-1
  cart2sph : MATLAB Function  TreatAsAtomicUnit=on
  r_ft : Outport
  az_rad : Outport  Port=2
  el_rad : Outport  Port=3
  rdot_ftps : Outport  Port=4
  True RAE : Outport  Port=5
  azdot_radps : Outport  Port=6
  eldot_radps : Outport  Port=7
  wires:
  cart2sph/8(K) -> Terminator1/1
  cart2sph/7(J) -> Terminator/1
  Demux2/3 -> cart2sph/6(zdot)
  Demux2/2 -> cart2sph/5(ydot)
  Demux2/1 -> cart2sph/4(xdot)
  Matrix Multiply1/1 -> Demux2/1
  Demux/1 -> cart2sph/1(x)
  Demux/2 -> cart2sph/2(y)
  Demux/3 -> cart2sph/3(z_d)
  Matrix Multiply/1 -> Demux/1
  Sum1/1 -> Matrix Multiply1/2
  Sum/1 -> Matrix Multiply/2
  T_N2F/1 -> Matrix Multiply/1, Matrix Multiply1/1
  Gain3/1 -> Mux/3
  Gain/1 -> Mux1/3
  Gain2/1 -> Mux2/3
  Gain1/1 -> Mux3/3
  Mux2/1 -> Sum1/2
  Mux3/1 -> Sum1/1
  Bus Selector2/2 -> Mux2/2  "<Edot_ftps>"
  Bus Selector2/1 -> Mux2/1  "<Ndot_ftps>"
  Bus Selector2/3 -> Gain2/1  "<hdot_ftps>"
  Own State Rate/1 -> Bus Selector2/1
  Intruder State Rate/1 -> Bus Selector3/1
  Bus Selector3/3 -> Gain1/1  "<hdot_ftps>"
  Mux/1 -> Sum/2
  Mux1/1 -> Sum/1
  Intruder State/1 -> Bus Selector1/1
  Bus Selector1/3 -> Gain/1  "<h_ft>"
  Bus Selector/2 -> Mux/2  "<e_ft>"
  Bus Selector/1 -> Mux/1  "<n_ft>"
  Bus Selector/3 -> Gain3/1  "<h_ft>"
  Own State/1 -> Bus Selector/1
  cart2sph/1(r) -> [range], r_ft/1, Bus Creator/1  "range"
  cart2sph/2(az_rad) -> Add1/2, Bus Creator/2  "az"
  cart2sph/3(el_rad) -> Add/2, Bus Creator/3  "el"
  Bus Creator/1 -> To Workspace/1, True RAE/1
  Bus Selector1/1 -> Mux1/1  "<n_ft>"
  Bus Selector1/2 -> Mux1/2  "<e_ft>"
  Bus Selector3/1 -> Mux3/1  "<Ndot_ftps>"
  Bus Selector3/2 -> Mux3/2  "<Edot_ftps>"
  Add1/1 -> az_rad/1, To Workspace1/1
  Add/1 -> el_rad/1, To Workspace2/1
  Divide1/1 -> Add/1
  Divide/1 -> Add1/1
  Colored Noise2/1(noisy) -> Divide1/1
  Colored Noise1/1(noisy) -> Divide/1
  cart2sph/4(rdot) -> rdot_ftps/1  "rdot"
  Colored Noise3/1(noisy) -> Divide2/1
  Colored Noise4/1(noisy) -> Divide3/1
  Divide2/1 -> Add2/1
  cart2sph/5(azdot_radps) -> To Workspace5/1, Add2/2  "azdot"
  cart2sph/6(eldot_radps) -> To Workspace6/1, Add3/2  "eldot"
  Divide3/1 -> Add3/1
  Add3/1 -> eldot_radps/1, To Workspace4/1
  Add2/1 -> azdot_radps/1, To Workspace3/1
  [range] -> Divide/2
  [range] -> Divide1/2
  [range] -> Divide2/2
  [range] -> Divide3/2

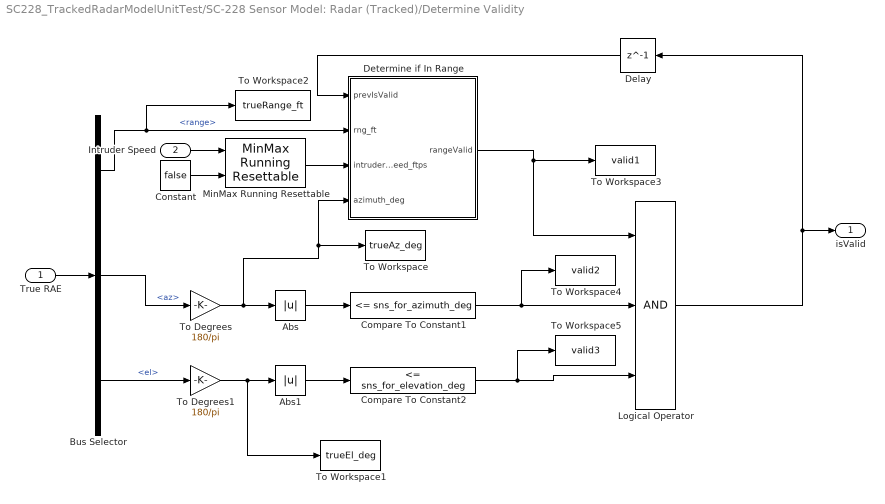
== system SC228_TrackedRadarModelUnitTest/SC-228 Sensor Model: Radar (Tracked)/Determine Validity ==
  True RAE : Inport
  Intruder Speed : Inport  Port=2
  Abs : Abs
  Abs1 : Abs
  Bus Selector : BusSelector  OutputSignals=range,az,el
  Compare To Constant1 : simulink/Logic and Bit Operations/Compare To Constant  relop=<=  const=sns_for_azimuth_deg  OutDataTypeStr=boolean
  Compare To Constant2 : simulink/Logic and Bit Operations/Compare To Constant  relop=<=  const=sns_for_elevation_deg  OutDataTypeStr=boolean
  Constant : Constant  Value=false
  Delay : Delay  DelayLength=1  InitialCondition=0
  Determine if In Range : Subsystem  mask{debugMode=debugMode}
      mask prompts: debugMode "Whether to run in Debug Mode with infinite detection range"
  Logical Operator : Logic  Inputs=3  AllPortsSameDT=off  OutDataTypeStr=boolean
  MinMax Running Resettable : simulink/Math Operations/MinMax Running Resettable  Function=max  vinit=0.0
  To Degrees : Gain  Gain=180/pi
  To Degrees1 : Gain  Gain=180/pi
  To Workspace : ToWorkspace  VariableName=trueAz_deg  SaveFormat=Timeseries  SampleTime=-1
  To Workspace1 : ToWorkspace  VariableName=trueEl_deg  SaveFormat=Timeseries  SampleTime=-1
  To Workspace2 : ToWorkspace  VariableName=trueRange_ft  SaveFormat=Timeseries  SampleTime=-1
  To Workspace3 : ToWorkspace  VariableName=valid1  SaveFormat=Timeseries  SampleTime=-1
  To Workspace4 : ToWorkspace  VariableName=valid2  SaveFormat=Timeseries  SampleTime=-1
  To Workspace5 : ToWorkspace  VariableName=valid3  SaveFormat=Timeseries  SampleTime=-1
  isValid : Outport
  wires:
  True RAE/1 -> Bus Selector/1
  Logical Operator/1 -> isValid/1, Delay/1
  Abs/1 -> Compare To Constant1/1
  Bus Selector/2 -> To Degrees/1  "<az>"
  Bus Selector/3 -> To Degrees1/1  "<el>"
  Abs1/1 -> Compare To Constant2/1
  Compare To Constant1/1 -> To Workspace4/1, Logical Operator/2
  Compare To Constant2/1 -> To Workspace5/1, Logical Operator/3
  To Degrees1/1 -> To Workspace1/1, Abs1/1
  Bus Selector/1 -> To Workspace2/1, Determine if In Range/2(rng_ft)  "<range>"
  Determine if In Range/1(rangeValid) -> Logical Operator/1, To Workspace3/1
  Intruder Speed/1 -> MinMax Running Resettable/1
  Constant/1 -> MinMax Running Resettable/2
  MinMax Running Resettable/1 -> Determine if In Range/3(intruderSpeed_ftps)
  To Degrees/1 -> To Workspace/1, Determine if In Range/4(azimuth_deg), Abs/1
  Delay/1 -> Determine if In Range/1(prevIsValid)

== system SC228_TrackedRadarModelUnitTest/AC1 - Track Following/Follow Trajectory/Compute Body Rates ==
  AircraftState : Inport
  Psi Dot : Inport  Port=2
  Theta Dot : Inport  Port=3
  Phi Dot : Inport  Port=4
  Bus Creator : BusCreator  Inputs=3
  Compute p : Subsystem
  Compute q : Subsystem
  Compute r : Subsystem
  p : Outport
  q : Outport  Port=2
  r : Outport  Port=3
  wires:
  Compute r/1(r) -> r/1
  Compute q/1(q) -> q/1
  Compute p/1(p) -> p/1
  Bus Creator/1 -> Compute p/2(Euler Rates), Compute q/2(Euler Rates), Compute r/2(Euler Rates)
  AircraftState/1 -> Compute p/1(State), Compute q/1(State), Compute r/1(State)
  Psi Dot/1 -> Bus Creator/1  "psidot"
  Phi Dot/1 -> Bus Creator/3  "phidot"
  Theta Dot/1 -> Bus Creator/2  "thetadot"

== system SC228_TrackedRadarModelUnitTest/AC1 - Track Following/Follow Trajectory/Compute Euler Angles ==
  AircraftState : Inport
  Constraints : Inport  Port=2
  Bus Selector : BusSelector  OutputSignals=psi_rad,theta_rad,phi_rad
  Bus Selector1 : BusSelector  OutputSignals=dphi_radps_max
  Discrete Derivative : simulink/Discrete/Discrete Derivative  gainval=1.0  ICPrevScaledInput=0.0  OutMin=[]  OutMax=[]  OutDataType=fixdt(1, 16)  OutScaling=2^-10  DoSatur=off
  Discrete Derivative1 : simulink/Discrete/Discrete Derivative  gainval=1.0  ICPrevScaledInput=0.0  OutMin=[]  OutMax=[]  OutDataType=fixdt(1, 16)  OutScaling=2^-10  DoSatur=off
  Discrete Derivative2 : simulink/Discrete/Discrete Derivative  gainval=1.0  ICPrevScaledInput=0.0  OutMin=[]  OutMax=[]  OutDataType=fixdt(1, 16)  OutScaling=2^-10  DoSatur=off
  IC : InitialCondition  Value=0
  IC1 : InitialCondition  Value=0
  IC2 : InitialCondition  Value=0
  Saturation Dynamic : simulink/Discontinuities/Saturation Dynamic  OutMin=[]  OutMax=[]  OutDataTypeStr=Inherit: Same as second input  OutDataType=fixdt(1, 16)  OutScaling=2^-10  DoSatur=off
  Unary Minus : UnaryMinus
  Psi Dot : Outport
  Theta Dot : Outport  Port=2
  "Phi Dot " : Outport  Port=3
  wires:
  Constraints/1 -> Bus Selector1/1
  IC2/1 -> Saturation Dynamic/2
  IC1/1 -> Theta Dot/1
  IC/1 -> Psi Dot/1
  Discrete Derivative2/1 -> IC2/1
  Discrete Derivative1/1 -> IC1/1
  Discrete Derivative/1 -> IC/1
  Bus Selector/3 -> Discrete Derivative2/1  "<phi_rad>"
  Bus Selector/2 -> Discrete Derivative1/1  "<theta_rad>"
  Bus Selector/1 -> Discrete Derivative/1  "<psi_rad>"
  AircraftState/1 -> Bus Selector/1
  Saturation Dynamic/1 -> "Phi Dot "/1
  Bus Selector1/1 -> Unary Minus/1, Saturation Dynamic/1  "<dphi_radps_max>"
  Unary Minus/1 -> Saturation Dynamic/3

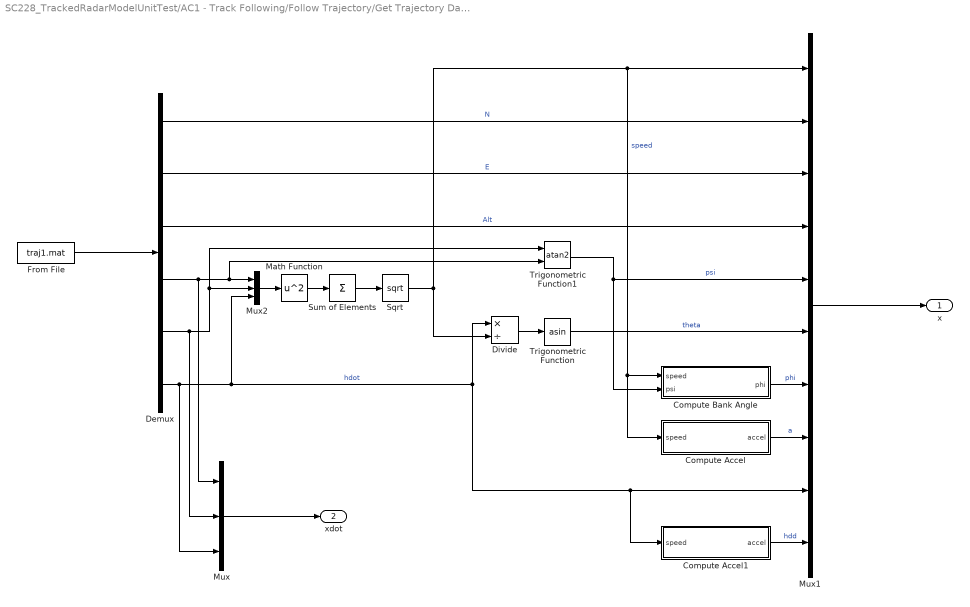
== system SC228_TrackedRadarModelUnitTest/AC1 - Track Following/Follow Trajectory/Get Trajectory Data ==
  Compute Accel : Subsystem
  Compute Accel1 : Subsystem
  Compute Bank Angle : Subsystem
  Demux : Demux  Outputs=6
  Divide : Product  Inputs=*/
  From File : FromFile  FileName=traj1.mat  SampleTime=0.1
  Math Function : Math  Operator=square  SaturateOnIntegerOverflow=on
  Mux : Mux  Inputs=3
  Mux1 : Mux  Inputs=10
  Mux2 : Mux  Inputs=3
  Sqrt : Sqrt  SaturateOnIntegerOverflow=on
  Sum of Elements : Sum  Inputs=+
  Trigonometric Function : Trigonometry  Operator=asin
  Trigonometric Function1 : Trigonometry  Operator=atan2
  x : Outport
  xdot : Outport  Port=2
  wires:
  Mux/1 -> xdot/1
  Compute Accel1/1(accel) -> Mux1/10  "hdd"
  Demux/5 -> Mux2/2, Trigonometric Function1/1, Mux/2
  Divide/1 -> Trigonometric Function/1
  Trigonometric Function1/1 -> Mux1/5, Compute Bank Angle/2(psi)  "psi"
  Trigonometric Function/1 -> Mux1/6  "theta"
  Compute Bank Angle/1(phi) -> Mux1/7  "phi"
  Compute Accel/1(accel) -> Mux1/8  "a"
  Mux1/1 -> x/1
  Sqrt/1 -> Divide/2, Mux1/1, Compute Bank Angle/1(speed), Compute Accel/1(speed)  "speed"
  Sum of Elements/1 -> Sqrt/1
  Math Function/1 -> Sum of Elements/1
  Mux2/1 -> Math Function/1
  Demux/6 -> Mux1/9, Compute Accel1/1(speed), Divide/1, Mux2/3, Mux/3  "hdot"
  Demux/4 -> Mux2/1, Trigonometric Function1/2, Mux/1
  Demux/3 -> Mux1/4  "Alt"
  Demux/2 -> Mux1/3  "E"
  Demux/1 -> Mux1/2  "N"
  From File/1 -> Demux/1

== system SC228_TrackedRadarModelUnitTest/AC1 - Track Following/Follow Trajectory/Null State Rate ==
  Bus Creator : BusCreator  Inputs='vdot_fpss','Ndot_ftps','Edot_ftps','hdot_ftps','psidot_radps','thetadot_radps','phidot_radps'  OutDataTypeStr=Bus: AircraftStateRate
  Constant{,1..6} (7 alike) : Constant  Value=0
  StateRate : Outport  OutDataTypeStr=Bus: AircraftStateRate
  wires:
  Constant6/1 -> Bus Creator/7  "phidot_radps"
  Constant5/1 -> Bus Creator/6  "thetadot_radps"
  Constant4/1 -> Bus Creator/5  "psidot_radps"
  Constant3/1 -> Bus Creator/4  "hdot_ftps"
  Constant2/1 -> Bus Creator/3  "Edot_ftps"
  Constant1/1 -> Bus Creator/2  "Ndot_ftps"
  Constant/1 -> Bus Creator/1  "vdot_fpss"
  Bus Creator/1 -> StateRate/1

== system SC228_TrackedRadarModelUnitTest/AC1 - Track Following/Follow Trajectory/Set LLA  ==
  State In : Inport
  Bus Assignment : BusAssignment  AssignedSignals=latLonAltState.lat_rad,latLonAltState.lon_rad,latLonAltState.dlat_radps,latLonAltState.dlon_radps,latLonAltState.alt_ft,latLonAltState.dalt_ftps
  Bus Selector : BusSelector  OutputSignals=e_ft,n_ft,h_ft,v_ftps,psi_rad,theta_rad
  Constant : Constant  Value=lat0
  Constant7 : Constant  Value=lon0
  Constant8 : Constant  Value=h0
  MATLAB Function : MATLAB Function  TreatAsAtomicUnit=on
  State Out : Outport
  wires:
  Bus Selector/6 -> MATLAB Function/6(theta_rad)  "<theta_rad>"
  Bus Selector/5 -> MATLAB Function/5(psi_rad)  "<psi_rad>"
  Bus Selector/4 -> MATLAB Function/4(v_ftps)  "<v_ftps>"
  Bus Selector/3 -> MATLAB Function/3(u_ft)  "<h_ft>"
  Bus Selector/2 -> MATLAB Function/2(n_ft)  "<n_ft>"
  Bus Selector/1 -> MATLAB Function/1(e_ft)  "<e_ft>"
  Constant8/1 -> MATLAB Function/9(h0)
  Constant7/1 -> MATLAB Function/8(lon0)
  Constant/1 -> MATLAB Function/7(lat0)
  State In/1 -> Bus Selector/1, Bus Assignment/1
  Bus Assignment/1 -> State Out/1
  MATLAB Function/6(dalt_ftps) -> Bus Assignment/7  "dalt_ftps"
  MATLAB Function/5(alt_ft) -> Bus Assignment/6  "alt_ft"
  MATLAB Function/4(dlon_radps) -> Bus Assignment/5  "dlon_radps"
  MATLAB Function/3(dlat_radps) -> Bus Assignment/4  "dlat_radps"
  MATLAB Function/2(lon_rad) -> Bus Assignment/3  "lon_rad"
  MATLAB Function/1(lat_rad) -> Bus Assignment/2  "lat_rad"

== system SC228_TrackedRadarModelUnitTest/AC1 - Track Following/Follow Trajectory/Set State ==
  x : Inport
  Bus Assignment : BusAssignment  AssignedSignals=v_ftps,n_ft,e_ft,h_ft,psi_rad,theta_rad,phi_rad,dv_ftps2,dh_ftps,ddh_ftps2
  Demux : Demux  Outputs=10
  Null AircraftState : Subsystem
  State : Outport
  wires:
  Demux/10 -> Bus Assignment/11
  Demux/9 -> Bus Assignment/10
  Bus Assignment/1 -> State/1
  Null AircraftState/1(State) -> Bus Assignment/1
  Demux/7 -> Bus Assignment/8  "phi"
  x/1 -> Demux/1
  Demux/6 -> Bus Assignment/7  "theta"
  Demux/5 -> Bus Assignment/6  "psi"
  Demux/4 -> Bus Assignment/5  "h"
  Demux/3 -> Bus Assignment/4  "E"
  Demux/2 -> Bus Assignment/3  "N"
  Demux/1 -> Bus Assignment/2  "v"
  Demux/8 -> Bus Assignment/9  "a"

== system SC228_TrackedRadarModelUnitTest/AC2 - Track Following/Follow Trajectory/Compute Body Rates ==
  AircraftState : Inport
  Psi Dot : Inport  Port=2
  Theta Dot : Inport  Port=3
  Phi Dot : Inport  Port=4
  Bus Creator : BusCreator  Inputs=3
  Compute p : Subsystem
  Compute q : Subsystem
  Compute r : Subsystem
  p : Outport
  q : Outport  Port=2
  r : Outport  Port=3
  wires:
  Compute r/1(r) -> r/1
  Compute q/1(q) -> q/1
  Compute p/1(p) -> p/1
  Bus Creator/1 -> Compute p/2(Euler Rates), Compute q/2(Euler Rates), Compute r/2(Euler Rates)
  AircraftState/1 -> Compute p/1(State), Compute q/1(State), Compute r/1(State)
  Psi Dot/1 -> Bus Creator/1  "psidot"
  Phi Dot/1 -> Bus Creator/3  "phidot"
  Theta Dot/1 -> Bus Creator/2  "thetadot"
